simulink model "test_find_circle"  (R2016b)
settings: Solver=VariableStepAuto  StartTime=0.0  StopTime=0.01  RelTol=1e-3
undefined symbols (not defined in the file or in its folder): Rec, SDTV
libraries: visionconversions x1, visiontextngfix x1, visionsources x1
settings Model: Creator=zeabus  LastModifiedBy=zeabus

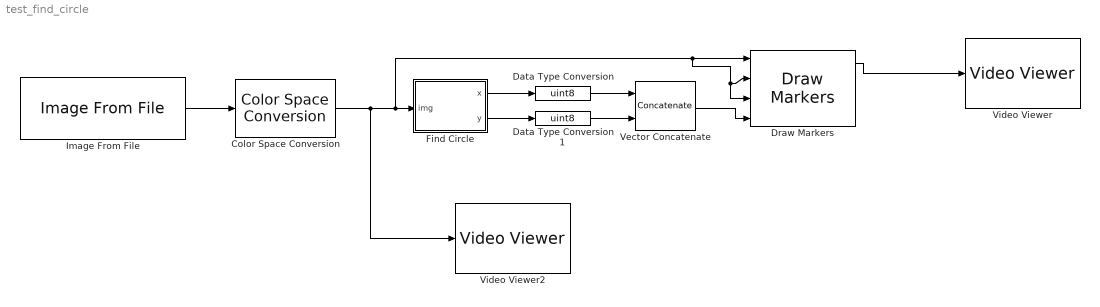
== system test_find_circle ==
  Color Space Conversion : visionconversions/Color Space  Conversion  conversion=Obsolete  conversionActive=R'G'B' to intensity  wp_str=D65  rec=Rec. 601 (SDTV)  sys=1125/60/2:1  imagePorts=One multidimensional signal
  Data Type Conversion : DataTypeConversion  OutDataTypeStr=uint8
  Data Type Conversion1 : DataTypeConversion  OutDataTypeStr=uint8
  Draw Markers : visiontextngfix/Draw Markers  shape=Circle  size=20  fill=on  fillClrSource=Specify via dialog  display=User-specified value  intensity=200  color=[0 0 255]  opacity=0.6  viewport=Entire image  antialiasing=off  inType=Obsolete  imagePorts=Separate color signals  prodOutputMode=Binary point scaling  prodOutputWordLength=32  prodOutputFracLength=14  memoryMode=Specify word length  memoryWordLength=16  memoryFracLength=14  roundingMode=Floor  overflowMode=off
  Find Circle : MATLAB Function  TreatAsAtomicUnit=on
  Image From File : visionsources/Image From File  Tag=vipblks_nd  FileName=C:\Users\zeabus\Desktop\Workspace\matlab\vision\images\imfindcircles0.png  imagePorts=One multidimensional signal  Ts=0.01  ImageDataType=Inherit from input image  Signed=on  WordLength=16  sdImageDataType=uint(8)  FractionLengthMode=User-defined  FractionLength=15  OutPortLabels=R|G|B
  Vector Concatenate : Concatenate  Mode=Multidimensional array
  Video Viewer : VideoViewer  FigPos=[822 681 560 404]
  Video Viewer2 : VideoViewer  FigPos=[255 659 560 404]
  wires:
  Find Circle/1(x) -> Data Type Conversion/1
  Find Circle/2(y) -> Data Type Conversion1/1
  Vector Concatenate/1 -> Draw Markers/4
  Data Type Conversion/1 -> Vector Concatenate/1
  Data Type Conversion1/1 -> Vector Concatenate/2
  Draw Markers/1 -> Video Viewer/1
  Image From File/1 -> Color Space Conversion/1
  Color Space Conversion/1 -> Video Viewer2/1, Draw Markers/2, Draw Markers/3, Draw Markers/1, Find Circle/1(img)

== matlab function test_find_circle/Find Circle ==
  data: img input; x output; y output
% Author : Supakit Kriangkhajorn,'Sensitivity',0.7
% Follow me : skconan
function [x,y]= findcircle(img)
    coder.extrinsic('imfindcircles'); 
    coder.extrinsic('isempty');
    coder.extrinsic('sortrows');
    coder.extrinsic('size');
    coder.extrinsic('gray2rgb');
    x = 150;
    y = 150;
    centerMax = [0,0];
    cols = 0;
    r = 0;
% gray = [img; img; img;];
%     img = img/10;
    im = img;
%     radiusMax = 0;
    status = 0;
    [centers, radius, metric] = imfindcircles(img,[10 60],'ObjectPolarity','bright','Sensitivity',0.85);
    circles = [centers, radius, metric];
   check = ~isempty(circles);
    if check
        status = 1;
        circles = sortrows(circles,3);
        [rows,cols] = size(circles);
        centerMax = circles(rows,1:2);
         radiusMax = circles(rows,3);
    end
         
x = round(centerMax(1));
y = round(centerMax(2));
